simulink model "Demo2"  (Simulink 6.5)
settings: Solver=FixedStepDiscrete  StartTime=0.0  StopTime=0.10  FixedStep=Ts  RelTol=1e-3  AbsTol=1e-3
PreLoadFcn:
  | assignin('base','Ts',[2e-6])
undefined symbols (not defined in the file): D1, Delta, powergui, Ts
libraries: powerlib x16, powerlib_extras x6
settings Model: Creator=sybille  LastModifiedBy=PC_0  ExtModeTrigMode=oneshot  ExtModeArmWhenConnect=off  ExtModeAutoUpdateStatusClock=off
settings DataIOCC: LimitDataPoints=off  SaveOutput=off  SaveTime=off  SignalLoggingName=sigsOut
settings OptimizationCC: BlockReduction=off  BooleanDataType=off  InlineInvariantSignals=on
settings DebuggingCC: CheckExecutionContextPreStartOutputMsg=on  CheckExecutionContextRuntimeOutputMsg=on  SolverPrmCheckMsg=none  MultiTaskDSMMsg=warning  MultiTaskCondExecSysMsg=none  StrictBusMsg=None
settings HardwareCC: TargetUnknown=on
settings RTWCC: IncludeERTFirstTime=on

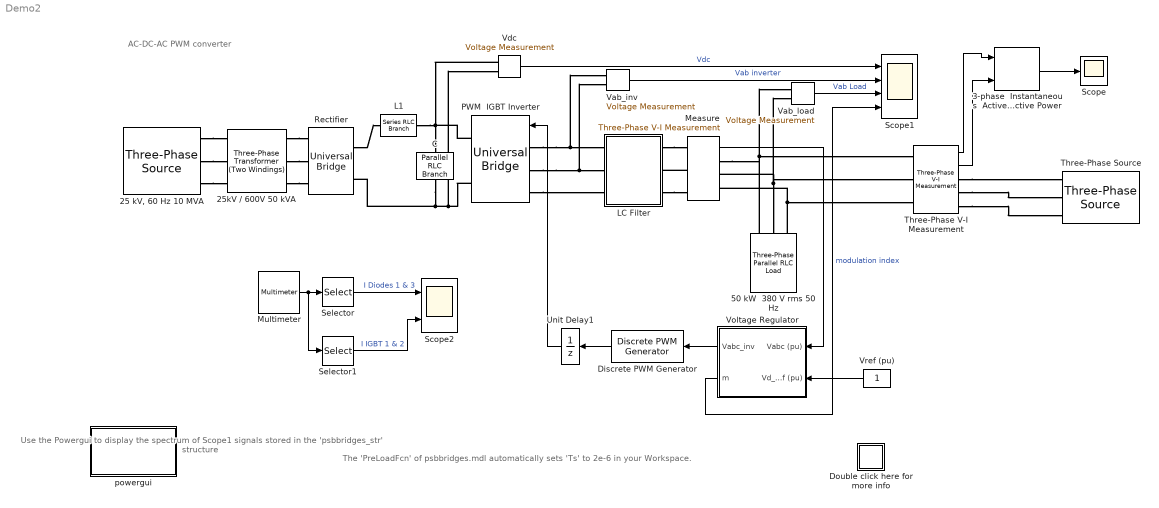
== system Demo2 ==
  note: AC-DC-AC PWM converter
  note: The 'PreLoadFcn' of psbbridges.mdl
      | automatically sets 'Ts' to 2e-6 in your Workspace.
  note: Use the Powergui to display
      | the spectrum of Scope1 signals
      | stored in the  'psbbridges_str'
      | structure
  "25 kV, 60 Hz 10 MVA" : powerlib/Electrical Sources/Three-Phase Source  DialogController=PMDialogs.PMDefaultMaskDlg  SystemSampleTime=-1  Voltage=25e3  PhaseAngle=0  Frequency=60  InternalConnection=Yg  SpecifyImpedance=on  Resistance=25e3^2/10e6/5  Inductance=25e3^2/10e6/377  ShortCircuitLevel=10e6  BaseVoltage=25e3  XRratio=5
  25kV / 600V 50 kVA : powerlib/Elements/Three-Phase Transformer (Two Windings)  DialogController=PMDialogs.PMDefaultMaskDlg  SystemSampleTime=-1  UNITS=pu  NominalPower=[ 50e3 , 60 ]  Winding1Connection=Yg  Winding1=[ 25e3 , 0.004 , 0.02 ]  Winding2Connection=Delta (D1)  Winding2=[ 600 , 0.004 , 0.02 ]  SetSaturation=off  Rm=200  Lm=200  Saturation="[ 0,0  ;  0.005,1.2  ;  1.0,1.4 ]"  Hysteresis=off  DataFile='hysteresis'  SetInitialFlux=off  InitialFluxes=[ 0.8 , -0.8 , 0.7 ]  Measurements=None  TransfoNumber=0  MoreParameters=off  BreakLoop=off  DataType=off
  3-phase  Instantaneous  Active & Reactive Power : powerlib_extras/Measurements/3-phase  Instantaneous  Active & Reactive Power  DialogController=PMDialogs.PMDefaultMaskDlg  SystemSampleTime=-1
  50 kW  380 V rms 50 Hz : powerlib/Elements/Three-Phase Parallel RLC Load  Orientation=down  DialogController=PMDialogs.PMDefaultMaskDlg  PhysicalDomain=powersysdomain  SubClassName=unknown  LeftPortType=p1  RightPortType=p1  LConnTagsString=A|B|C  Configuration=Y (grounded)  NominalVoltage=380  NominalFrequency=50  ActivePower=50e3  InductivePower=0  CapacitivePower=0  Measurements=None
  C : powerlib/Elements/Parallel RLC Branch  Orientation=down  DialogController=PMDialogs.PMDefaultMaskDlg  PhysicalDomain=powersysdomain  SubClassName=unknown  LeftPortType=p1  RightPortType=p1  LConnTagsString=a  RConnTagsString=__new0  BranchType=C  Resistance=1.0  Inductance=1.0  SetiL0=off  InitialCurrent=0  Capacitance=5000e-06  Setx0=off  InitialVoltage=0  Measurements=None
  Discrete PWM Generator : powerlib_extras/Discrete  Control Blocks/Discrete PWM Generator  Orientation=left  DialogController=PMDialogs.PMDefaultMaskDlg  SystemSampleTime=-1  GeneratorMode="3-arm  bridge (6 pulses)"  Fc=2000  Ts=Ts  Internal=off  mIndex=0.4  Freq=60  Phase=0
  Double click here for more info : Subsystem
      settings: OpenFcn=showdemo(bdroot(gcb))
      mask Display: disp('?')
  L1 : powerlib/Elements/Series RLC Branch  DialogController=PMDialogs.PMDefaultMaskDlg  PhysicalDomain=powersysdomain  SubClassName=unknown  LeftPortType=p1  RightPortType=p1  LConnTagsString=__new0  RConnTagsString=__new0  BranchType=L  Resistance=1.0  Inductance=200e-6  SetiL0=off  InitialCurrent=0  Capacitance=1.0  Setx0=off  InitialVoltage=0  Measurements=None
  LC Filter : Subsystem
  Measure : powerlib/Measurements/Three-Phase V-I Measurement  DialogController=PMDialogs.PMDefaultMaskDlg  SystemSampleTime=-1  VoltageMeasurement=phase-to-ground  SetLabelV=off  LabelV=V1  Vpu=on  CurrentMeasurement=no  SetLabelI=off  LabelI=I1  Ipu=off  Pbase=1e3  Vbase=380  OutputType=Magnitude  PhasorSimulation=off  PSBequivalent=0
  Multimeter : powerlib/Measurements/Multimeter  Tag=PoWeRsYsTeMmEaSuReMeNt  SystemSampleTime=-1  PhasorSimulation=off  OutputType=Magnitude  sel=[1 3 7 8]  L=12  Gain=[1 1 1 1]  yselected="{'Isw1: Rectifier','Isw3: Rectifier','Isw1: PWM  IGBT Inverter','Isw2: PWM  IGBT Inverter'};"  PSBOutputType=1  PSBequivalent=0  AxesSetting=[0,0.1,-100,100]  Display=0  SavedBlockNames=-11
      settings: AttributesFormatString=\n
  PWM  IGBT Inverter : powerlib/Power Electronics/Universal Bridge  Orientation=left  DialogController=PMDialogs.PMDefaultMaskDlg  SystemSampleTime=-1  Arms=3  SnubberResistance=5000  SnubberCapacitance=inf  Device=IGBT / Diodes  Ron=1e-3  Lon=0  ForwardVoltages="[  0.0  0.0  ]"  ForwardVoltage=.8  GTOparameters=[ 1e-6 ,1e-6 ]  IGBTparameters=[ 1e-6 , 2e-6 ]  Measurements=Device currents  converterType=Rectifier
  Rectifier : powerlib/Power Electronics/Universal Bridge  DialogController=PMDialogs.PMDefaultMaskDlg  SystemSampleTime=-1  Arms=3  SnubberResistance=100  SnubberCapacitance=0.1e-6  Device=Diodes  Ron=1e-3  Lon=0  ForwardVoltages="[  0.8  0.8  ]"  ForwardVoltage=.8  GTOparameters=[ 10e-6 , 20e-6 ]  IGBTparameters=[ 1e-6 , 2e-6 ]  Measurements=Device currents  converterType=Rectifier
  Scope : Scope
      settings: MaxDataPoints=10000000  SampleInput=on  SampleTime=10e-6
  Scope1 : Scope  NumInputPorts=4
      settings: TimeRange=0.1  YMin=0~-1500~-750~0.4  YMax=1100~1500~750~1.1  SaveName=psbbridges_str
  Scope2 : Scope  NumInputPorts=2
      settings: TimeRange=0.09999999999999999  YMin=-10~-125  YMax=100~125
  Selector : Selector  InputType=Vector  ElementSrc=Internal  Elements=[1 2]  RowSrc=Internal  Rows=1  ColumnSrc=Internal  Columns=1  InputPortWidth=4  IndexIsStartValue=off
  Selector1 : Selector  InputType=Vector  ElementSrc=Internal  Elements=[3 4]  RowSrc=Internal  Rows=1  ColumnSrc=Internal  Columns=1  InputPortWidth=4  IndexIsStartValue=off
  Three-Phase V-I Measurement : powerlib/Measurements/Three-Phase V-I Measurement  DialogController=PMDialogs.PMDefaultMaskDlg  SystemSampleTime=-1  VoltageMeasurement=phase-to-ground  SetLabelV=off  LabelV=Vabc  Vpu=off  CurrentMeasurement=yes  SetLabelI=off  LabelI=Iabc  Ipu=off  Pbase=100e6  Vbase=500e3  OutputType=Complex  PhasorSimulation=off  PSBequivalent=0
  Three-Phase Source : powerlib/Electrical Sources/Three-Phase Source  Orientation=left  DialogController=PMDialogs.PMDefaultMaskDlg  SystemSampleTime=-1  Voltage=380  PhaseAngle=0  Frequency=50  InternalConnection=Yg  SpecifyImpedance=off  Resistance=0.001  Inductance=0.001  ShortCircuitLevel=100e6  BaseVoltage=25e3  XRratio=7
  Unit Delay1 : UnitDelay  Orientation=left  SampleTime=Ts
  Vab_inv : powerlib/Measurements/Voltage Measurement  Tag=PoWeRsYsTeMmEaSuReMeNt  DialogController=PMDialogs.PMDefaultMaskDlg  SystemSampleTime=-1  PhasorSimulation=off  OutputType=Magnitude  PSBequivalent=0
  Vab_load : powerlib/Measurements/Voltage Measurement  Tag=PoWeRsYsTeMmEaSuReMeNt  DialogController=PMDialogs.PMDefaultMaskDlg  SystemSampleTime=-1  PhasorSimulation=off  OutputType=Magnitude  PSBequivalent=0
  Vdc : powerlib/Measurements/Voltage Measurement  Tag=PoWeRsYsTeMmEaSuReMeNt  DialogController=PMDialogs.PMDefaultMaskDlg  SystemSampleTime=-1  PhasorSimulation=off  OutputType=Magnitude  PSBequivalent=0
  Voltage Regulator : Subsystem  Orientation=left  mask( Voltage Regulator){Kp=0.4, Ki=500, Ts=Ts}
      mask prompts: Kp "Proportional gain  Kp:"; Ki "Integral gain Ki:"; Ts "Sample time (s) :"
  "Vref (pu) " : Constant  Orientation=left  Value=1  OutDataType=sfix(16)  ConRadixGroup=Use specified scaling  OutScaling=2^0  SampleTime=inf  FramePeriod=inf
  powergui : Subsystem  Priority=2  AncestorBlock=powerlib/powergui  InitFcn=powergui( 'InitFcn_Callback' , gcb , 0 , [ ] );  mask(PSB option menu block){SimulationMode=Discrete, SampleTime=Ts, echomessages=on, RestoreLinks=warning, x0status=blocks, Frange=[0:2:500], Ylog=off, Xlog=on, ShowGrid=off, save=off, variable=ZData, structure=psbbridges_str, ZoomFFT=on, StartTime=0.1-2/50, cycles=2, DisplayStyle=off, fundamental=50, FreqAxis=off, MaxFrequency=7000, frequencyindice=60, frequencyindicesteady=1, RmsSteady=1, display=off, Ts=0, frequency=60, methode=off, HookPort=off, Interpol=off}
      mask prompts: SimulationMode "Simulation mode"; SampleTime "Sample time Ts (when simulation mode is Discrete) (s)"; echomessages "Echo  Messages"; RestoreLinks "Restore disabled links"; x0status "Initial electrical states status"; Frange "Impedance tool: Frequency Range"; Ylog "Impedance tool: Log impedance"; Xlog "Impedance tool: log Frequency"; ShowGrid "Impedance tool: grid"; save "Impedance tool: Save Data To Workspace"; variable "Impedance tool: Variable Name"; structure "Structure Name (PSBFFTSCOPE)"; ZoomFFT "ZoomFFT (PSBFFTSCOPE)"; StartTime "Start Time (PSBFFTSCOPE)"; cycles "Cycles (PSBFFTSCOPE)"; DisplayStyle "Display style (PSBFFTSCOPE)"; fundamental "Fundamental (PSBFFTSCOPE)"; FreqAxis "Frequency Axis (PSBFFTSCOPE)"; MaxFrequency "Max Frequency (PSBFFTSCOPE)"; frequencyindice "Load flow frequency (Hz)"; frequencyindicesteady "Frequency indice (STEADYSTATE)"; RmsSteady "RMS display (STEADYSTATE)"; display "Display Results"; Ts "OBSOLETE 1"; frequency "Phasor frequency (Hz)"; methode "Phasor simulation"; HookPort "Hook port"; Interpol "Interpolate"
      mask init:
      | powerlibroot = which('powersysdomain');
      | PSBroot = powerlibroot(1:end-16);
      | %
      | switch SimulationMode
      | 	case 1
      | 		message=sprintf('Continuous');
      | 	case 2
      |         SampleTimeeval=evalin('base',SampleTime,'NaN');
      |         if isnan(SampleTimeeval)
      |             message=sprintf('Warning !!,\nUndefined sample time');
      |         else
      |             message=sprintf('Discrete,\nTs = %.4g s.',SampleTimeeval);
      |         end
      | 	case 3
      | 		message=sprintf('Phasors');
      | end
      | if strcmp(bdroot,'powerlib')
      |   message='powergui';
      | end
      | power_initmask();
      settings: CopyFcn=powergui( 'Copy_Callback' , gcb , 0 , [ ] );  ModelCloseFcn=powergui( 'CloseButton_Callback' , gcb , [ ] , [ ] );  PreSaveFcn=powergui( 'CloseButton_Callback' , gcb , [ ] , [ ] );  NameChangeFcn=powergui( 'NameChangeFcn_Callback' , gcb , 0 , [ ] );
      settings: DeleteFcn=|
      | powergui( 'Copy_Callback' , gcb , 1 , [ ] );
      | powergui( 'CloseButton_Callback' , gcb , [ ] , [ ] );
      settings: OpenFcn=|
      | if (power_openblockproxy ('secondary'))
      | powergui(gcb,'PM')
      | end;
      mask Help: web(psbhelp)
      mask StyleString: popup(Continuous|Discrete|Phasor),edit,checkbox,popup(yes|warning|no),popup(blocks|steady|zero),edit,checkbox,checkbox,checkbox,checkbox,edit,edit,checkbox,edit,edit,edit,edit,checkbox,edit,edit,edit,edit,checkbox,edit,edit,checkbox,checkbox,checkbox
      mask CallbackString: ||||||||||||||||||||||||||powergui('HookPort',[],[],gcb);|
      mask Display: disp(message)
  wires:
  "Vref (pu) "/1 -> Voltage Regulator/2(Vd_ref (pu))
  Selector/1 -> Scope2/1  "I Diodes 1 & 3"
  Selector1/1 -> Scope2/2  "I IGBT 1 & 2"
  Discrete PWM Generator/1 -> Unit Delay1/1
  Voltage Regulator/1(Vabc_inv) -> Discrete PWM Generator/1
  Voltage Regulator/2(m) -> Scope1/4  "modulation index"
  Multimeter/1 -> Selector/1, Selector1/1
  Vdc/1 -> Scope1/1  "Vdc"
  Vab_load/1 -> Scope1/3  "Vab Load"
  Vab_inv/1 -> Scope1/2  "Vab inverter"
  Unit Delay1/1 -> PWM  IGBT Inverter/1
  Measure/1 -> Voltage Regulator/1(Vabc (pu))
  Three-Phase V-I Measurement/1 -> 3-phase  Instantaneous  Active & Reactive Power/1
  Three-Phase V-I Measurement/2 -> 3-phase  Instantaneous  Active & Reactive Power/2
  3-phase  Instantaneous  Active & Reactive Power/1 -> Scope/1
  connections:
  PWM  IGBT Inverter/RConn2 -- C/RConn1 -- Rectifier/RConn2 -- Vdc/LConn2
  Vdc/LConn1 -- C/LConn1 -- L1/RConn1 -- PWM  IGBT Inverter/RConn1
  25kV / 600V 50 kVA/RConn3 -- Rectifier/LConn3
  "25 kV, 60 Hz 10 MVA"/RConn1 -- 25kV / 600V 50 kVA/LConn1
  "25 kV, 60 Hz 10 MVA"/RConn2 -- 25kV / 600V 50 kVA/LConn2
  "25 kV, 60 Hz 10 MVA"/RConn3 -- 25kV / 600V 50 kVA/LConn3
  25kV / 600V 50 kVA/RConn2 -- Rectifier/LConn2
  LC Filter/RConn1 -- Measure/LConn1
  Measure/LConn2 -- LC Filter/RConn2
  LC Filter/RConn3 -- Measure/LConn3
  25kV / 600V 50 kVA/RConn1 -- Rectifier/LConn1
  Rectifier/RConn1 -- L1/LConn1
  PWM  IGBT Inverter/LConn2 -- LC Filter/LConn2 -- Vab_inv/LConn2
  PWM  IGBT Inverter/LConn3 -- LC Filter/LConn3
  PWM  IGBT Inverter/LConn1 -- LC Filter/LConn1 -- Vab_inv/LConn1
  Measure/RConn2 -- Vab_load/LConn2 -- 50 kW  380 V rms 50 Hz/LConn2 -- Three-Phase V-I Measurement/LConn2
  Measure/RConn1 -- 50 kW  380 V rms 50 Hz/LConn1 -- Vab_load/LConn1 -- Three-Phase V-I Measurement/LConn1
  50 kW  380 V rms 50 Hz/LConn3 -- Measure/RConn3 -- Three-Phase V-I Measurement/LConn3
  Three-Phase V-I Measurement/RConn1 -- Three-Phase Source/RConn1
  Three-Phase V-I Measurement/RConn2 -- Three-Phase Source/RConn2
  Three-Phase V-I Measurement/RConn3 -- Three-Phase Source/RConn3

== system Demo2/Double click here for more info ==
  note: This example of AC-DC-AC converter illustrates use of Universal Bridge,
      | Multimeter, and Powergui  blocks, as well as discrete control blocks of the Extras library
  note: Circuit Description
  note: Demonstration
  note: A  60 Hz, voltage source feeds a 50 Hz, 50 kW load through an  AC-DC-AC  converter.
      |
      | The 600V, 60 Hz voltage obtained at secondary of the Wye/Delta transformer is first rectified by a six pulse diode bridge.
      | The filtered DC voltage is applied to an IGBT two-level inverter generating 50 Hz.
      | The IGBT inverter uses Pulse Width Modulation (PWM) at a 2 kHz carrier frequency.
      | The circuit is discretized at a sample time of 2 us
      |
      | The load voltage is regulated at 1 pu (380 V rms) by a PI voltage regulator using abc_to_dq and dq_to_abc transfomations.
      | The first output of the voltage regulator is a vector containing the three modulating signals used by the PMW Generator
      | to generate the 6 IGBT pulses. The second output returns the modulation index.
      |
      | The Discrete 3-Phase PWM Pulse Generator is available in the Extras/Discrete Control Blocks library.
      | The voltage regulator has been  built from blocks of the Extras/Measurements and Extras/ Discrete Control libraries
      |
      | The Multimeter block is used to observe diode and IGBT currents.
      | In order to allow further signal processing, signals displayed on  Scope1 block  (sampled at simulation sampling rate of 2us )
      | are stored in a  variable named 'psbbridges_str' (structure with time) .
  note: Start the simulation. After a transient period of approximately  50 ms, the system reaches a steady state.
      | Observe  voltage waveforms at  DC bus, inverter output  and load on Scope1.
      | The harmonics generated by the inverter around around multiples of 2 kHz are filtered by the  LC filter.
      |
      | As expected the peak value of the load voltage is 537 V (380 Vrms).
      | In steady state, the mean value of the modulation index is m = 0.80 and the mean value of the  DC  voltage is 778 V.
      | The fundamental component of 50 Hz voltage burried in the chopped inverter voltage is therefore:
      | Vab = 778 V * 0.612 * 0.80 = 381 V rms
      |
      | Once  simulation is completed, open the Powergui and select  'FFT Analysis' to display the 0 - 7000 Hz frequency spectrum of signals saved
      | in the 'psbbridges_str' structure. The FFT will be performed on  a 2-cycle window starting at t=0.1-2/50 (last 2 cycles of recording).
      | Select input labeled 'Vab Load' . Click on Display and observe the frequency spectrum of last 2 cycles.
      | Notice harmonics around multiples of the 2 kHz carrier frequency. Maximum harmonic is 1.4 % of fundamental and THD is 2%.
      |
      | Observe diode currents on trace 1 of Scope2, showing commutation from  diode 1 to diode 3.  Also observe on trace 2 currents in
      | switches 1 and 2 of the IGBT/Diode bridge (upper and lower switches connected to phase A). These two currents are complementary.
      | A positive current indicates a current flowing in the IGBT, whereas a negative current indicates a current flowing in the antiparallel diode.
  note: G. Sybille (Hydro-Quebec)

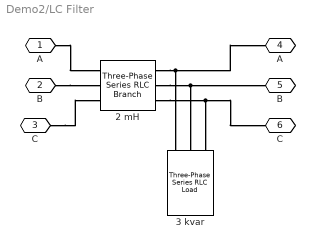
== system Demo2/LC Filter ==
  "2 mH " : powerlib/Elements/Three-Phase Series RLC Branch  DialogController=PMDialogs.PMDefaultMaskDlg  PhysicalDomain=powersysdomain  SubClassName=unknown  LeftPortType=p1  RightPortType=p1  LConnTagsString=A|B|C  RConnTagsString=A|B|C  BranchType=L  Resistance=1.0  Inductance=2e-3  Capacitance=1.0  Measurements=None
  3 kvar : powerlib/Elements/Three-Phase Series RLC Load  Orientation=down  DialogController=PMDialogs.PMDefaultMaskDlg  PhysicalDomain=powersysdomain  SubClassName=unknown  LeftPortType=p1  RightPortType=p1  LConnTagsString=A|B|C  Configuration=Y (grounded)  NominalVoltage=380  NominalFrequency=50  ActivePower=0  InductivePower=0  CapacitivePower=3e3  Measurements=None
  A : PMIOPort  Port=1  Side=Left
  B : PMIOPort  Port=2  Side=Left
  C : PMIOPort  Port=3  Side=Left
  "A " : PMIOPort  Orientation=left  Port=4  Side=Right
  "B " : PMIOPort  Orientation=left  Port=5  Side=Right
  "C " : PMIOPort  Orientation=left  Port=6  Side=Right
  connections:
  B/RConn1 -- "2 mH "/LConn2
  A/RConn1 -- "2 mH "/LConn1
  C/RConn1 -- "2 mH "/LConn3
  "2 mH "/RConn1 -- "A "/RConn1 -- 3 kvar/LConn1
  "2 mH "/RConn2 -- "B "/RConn1 -- 3 kvar/LConn2
  "2 mH "/RConn3 -- "C "/RConn1 -- 3 kvar/LConn3

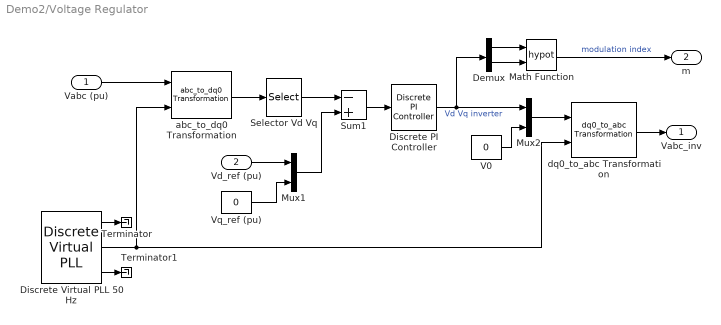
== system Demo2/Voltage Regulator ==
  Vabc (pu) : Inport
  Vd_ref (pu) : Inport  Port=2
  Demux : Demux  Outputs=2
  Discrete PI Controller : powerlib_extras/Discrete  Control Blocks/Discrete PI Controller  DialogController=PMDialogs.PMDefaultMaskDlg  SystemSampleTime=-1  Kp=Kp  Ki=Ki  Par_Limits=[1 -1]  Init=0  Ts=Ts
  Discrete Virtual PLL 50 Hz : powerlib_extras/Discrete  Control Blocks/Discrete Virtual PLL  DialogController=PMDialogs.PMDefaultMaskDlg  SystemSampleTime=-1  Freq=50  Phase=0  Ts=Ts
  Math Function : Math  Operator=hypot  SaturateOnIntegerOverflow=on
  Mux1 : Mux  Inputs=2
  Mux2 : Mux  Inputs=2
  Selector Vd Vq : Selector  InputType=Vector  ElementSrc=Internal  Elements=[1 2]  RowSrc=Internal  Rows=1  ColumnSrc=Internal  Columns=1  InputPortWidth=3  IndexIsStartValue=off
  Sum1 : Sum  Inputs=-+  SaturateOnIntegerOverflow=on  InputSameDT=on
  Terminator : Terminator
  Terminator1 : Terminator
  V0 : Constant  Value=0  OutDataType=sfix(16)  ConRadixGroup=Use specified scaling  OutScaling=2^0  SampleTime=inf  FramePeriod=inf
  Vq_ref (pu) : Constant  Value=0  OutDataType=sfix(16)  ConRadixGroup=Use specified scaling  OutScaling=2^0  SampleTime=inf  FramePeriod=inf
  abc_to_dq0 Transformation : powerlib_extras/Measurements/abc_to_dq0 Transformation  DialogController=PMDialogs.PMDefaultMaskDlg  SystemSampleTime=-1
  dq0_to_abc Transformation : powerlib_extras/Measurements/dq0_to_abc Transformation  DialogController=PMDialogs.PMDefaultMaskDlg  SystemSampleTime=-1
  Vabc_inv : Outport
  m : Outport  Port=2
  wires:
  abc_to_dq0 Transformation/1 -> Selector Vd Vq/1
  Vabc (pu)/1 -> abc_to_dq0 Transformation/1
  Selector Vd Vq/1 -> Sum1/1
  Sum1/1 -> Discrete PI Controller/1
  Mux2/1 -> dq0_to_abc Transformation/1
  V0/1 -> Mux2/2
  dq0_to_abc Transformation/1 -> Vabc_inv/1
  Discrete Virtual PLL 50 Hz/2 -> abc_to_dq0 Transformation/2, dq0_to_abc Transformation/2
  Vd_ref (pu)/1 -> Mux1/1
  Vq_ref (pu)/1 -> Mux1/2
  Mux1/1 -> Sum1/2
  Discrete Virtual PLL 50 Hz/1 -> Terminator/1
  Discrete Virtual PLL 50 Hz/3 -> Terminator1/1
  Discrete PI Controller/1 -> Demux/1, Mux2/1  "Vd Vq inverter"
  Demux/1 -> Math Function/1
  Demux/2 -> Math Function/2
  Math Function/1 -> m/1  "modulation index"

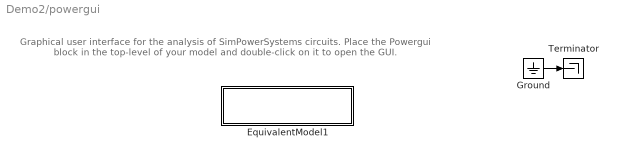
== system Demo2/powergui ==
  note: Graphical user interface for the analysis of  SimPowerSystems circuits.
      | Place the Powergui block in the top-level of your model and double-click
      | on it to open the GUI.
  EquivalentModel1 : Subsystem
      mask init:
      | SPS = get_param(gcbh,'UserData');
      | if isempty(SPS)
      | 	Ts=1;
      |     A=0;
      |     B=0;
      |     C=0;
      |     D=0;
      |     x0=0;
      |     SwitchResistance=1;
      |     SwitchType=1;
      |     SwitchGateInitialValue=1;
      |     OutputsToResetToZero=1;
      | else
      | 	Ts=SPS.PowerguiInfo.Ts;
      | 	A=SPS.Adiscrete;
      |     B=SPS.Bdiscrete;
      |     C=SPS.Cdiscrete;
      |     D=SPS.Ddiscrete;
      |     x0=SPS.x0discrete;
      |     SwitchResistance=SPS.SwitchResistance;
      |     SwitchType=SPS.SwitchType;
      |     SwitchGateInitialValue=SPS.SwitchGateInitialValue;
      |     OutputsToResetToZero=SPS.YSwitchCurrent;
      | end
      mask Display:
      | color('orange')
      | disp('EQUIVALENT CIRCUIT')
  Ground : Ground
  Terminator : Terminator
  wires:
  Ground/1 -> Terminator/1

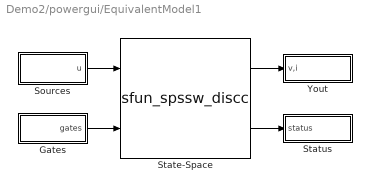
== system Demo2/powergui/EquivalentModel1 ==
  Gates : Subsystem
  Sources : Subsystem
  State-Space : S-Function  FunctionName=sfun_spssw_discc  Parameters=Ts,A, B, C, D, x0, SwitchResistance ,SwitchType, SwitchGateInitialValue, OutputsToResetToZero
  Status : Subsystem
  Yout : Subsystem
  wires:
  State-Space/1 -> Yout/1(v,i)
  State-Space/2 -> Status/1(status)
  Sources/1(u) -> State-Space/1
  Gates/1(gates) -> State-Space/2

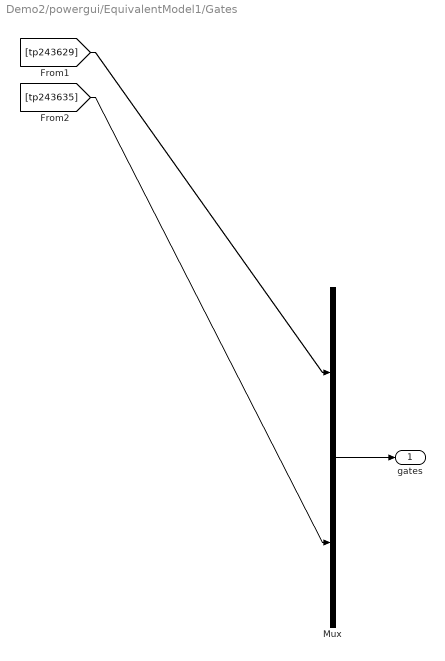
== system Demo2/powergui/EquivalentModel1/Gates ==
  Mux : Mux  Inputs=[6 6]
  gates : Outport
  wires:
  Mux/1 -> gates/1
  [tp243629] -> Mux/1
  [tp243635] -> Mux/2

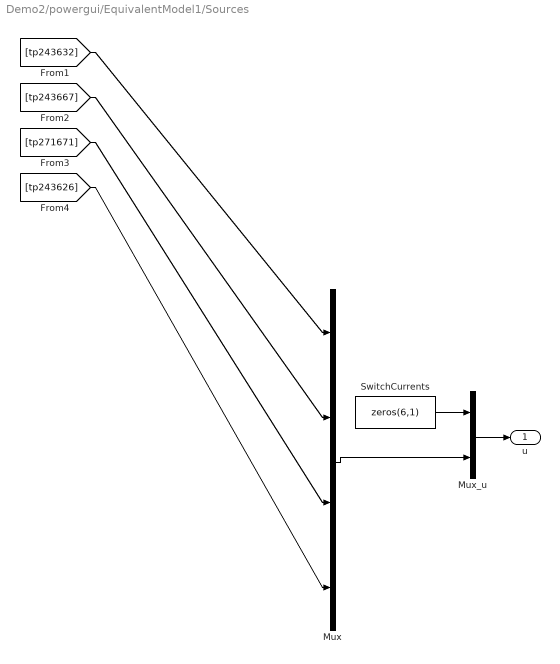
== system Demo2/powergui/EquivalentModel1/Sources ==
  Mux : Mux  Inputs=[6 3 3 6]
  Mux_u : Mux  Inputs=[6 18]
  SwitchCurrents : Constant  Value=zeros(6,1)  OutDataType=sfix(16)  ConRadixGroup=Use specified scaling  OutScaling=2^0  SampleTime=inf  FramePeriod=inf
  u : Outport
  wires:
  Mux/1 -> Mux_u/2
  SwitchCurrents/1 -> Mux_u/1
  Mux_u/1 -> u/1
  [tp243632] -> Mux/1
  [tp243667] -> Mux/2
  [tp271671] -> Mux/3
  [tp243626] -> Mux/4

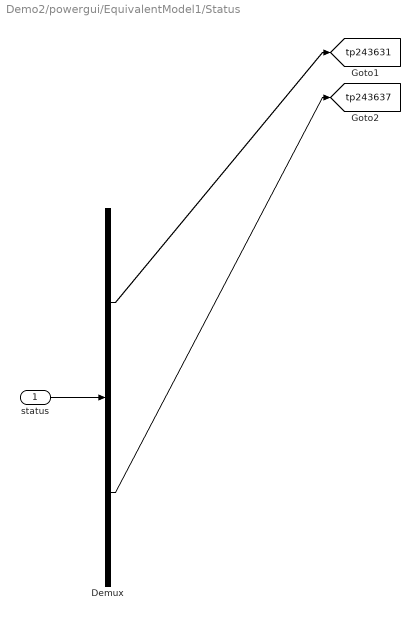
== system Demo2/powergui/EquivalentModel1/Status ==
  status : Inport
  Demux : Demux  Outputs=[6 6]
  tag scope: tp243631=global, tp243637=global
  wires:
  status/1 -> Demux/1
  Demux/1 -> [tp243631]
  Demux/2 -> [tp243637]

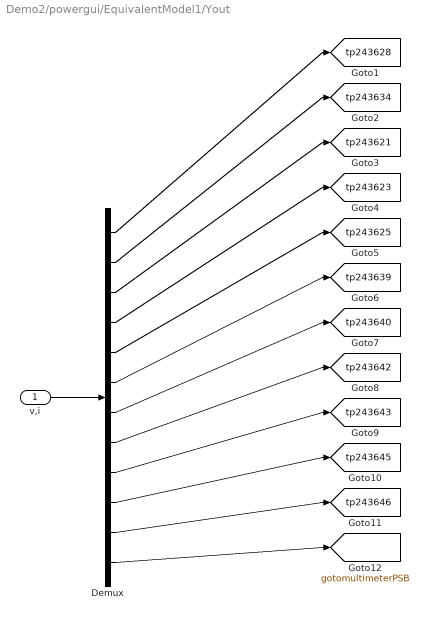
== system Demo2/powergui/EquivalentModel1/Yout ==
  v,i : Inport
  Demux : Demux  Outputs=[6 6 1 1 1 1 1 1 1 1 1 12]
  tag scope: gotomultimeterPSB=global, tp243621=global, tp243623=global, tp243625=global, tp243628=global, tp243634=global, tp243639=global, tp243640=global, tp243642=global, tp243643=global, tp243645=global, tp243646=global
  wires:
  v,i/1 -> Demux/1
  Demux/1 -> [tp243628]
  Demux/2 -> [tp243634]
  Demux/3 -> [tp243621]
  Demux/4 -> [tp243623]
  Demux/5 -> [tp243625]
  Demux/6 -> [tp243639]
  Demux/7 -> [tp243640]
  Demux/8 -> [tp243642]
  Demux/9 -> [tp243643]
  Demux/10 -> [tp243645]
  Demux/11 -> [tp243646]
  Demux/12 -> [gotomultimeterPSB]
